simulink model "test"  (R2022b)
settings: Solver=VariableStepAuto  StartTime=0.0  StopTime=10.0  RelTol=1e-3
model workspace (MAT data in the model file):
  Var = 1
  sta = Simulink.Signal
  sta.DataType = 'Bus: Geskf_Res'
  sta.Dimensions = -1
  sta.DimensionsMode = 'auto'
  sta.Complexity = 'auto'
  sta.SampleTime = -1
  sta.SamplingMode = 'auto'
values from neighbouring files (symbols this model uses):
  a = [x1 x2]    [jocobi_test.m]
undefined symbols (not defined in the file or in its folder): stb
settings Model: Creator=89565  LastModifiedBy=89565

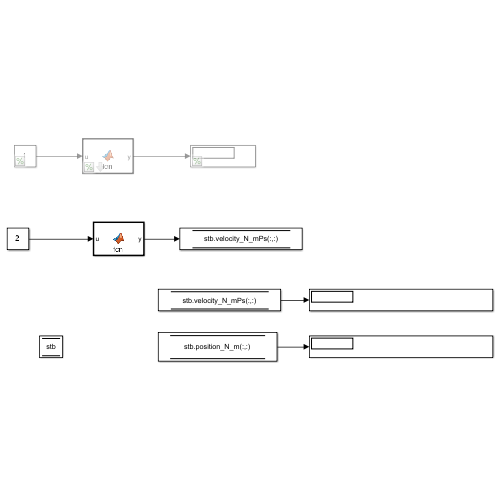
[thumbnail: Simulink's stored preview of the top-level diagram]
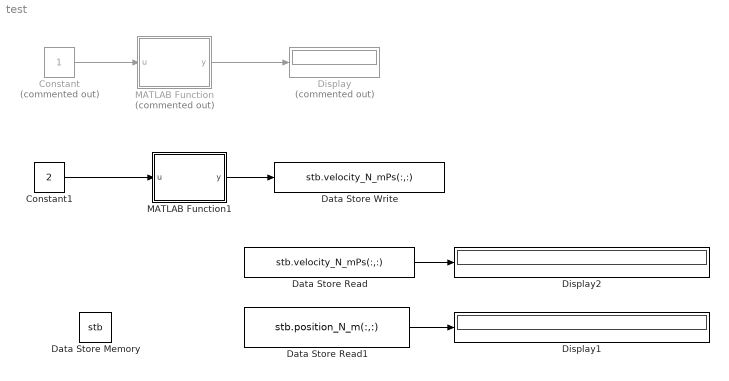
== system test ==
  Constant : Constant  Commented=on
  Constant1 : Constant  Value=2  OutDataTypeStr=double
  Data Store Read : DataStoreRead  DataStoreName=stb  DataStoreElements=stb.velocity_N_mPs(:,:)  IndexOptions=Index vector (dialog)  Indices=1  OutputSizes=1
  Data Store Read1 : DataStoreRead  DataStoreName=stb  DataStoreElements=stb.position_N_m(:,:)  IndexOptions=Index vector (dialog)  Indices=1  OutputSizes=1
  Data Store Write : DataStoreWrite  DataStoreName=stb  DataStoreElements=stb.velocity_N_mPs(:,:)  IndexOptions=Index vector (dialog)  Indices=1  OutputSizes=1
  Data Store Memory : DataStoreMemory  DataStoreName=stb  WriteAfterWriteMsg=warning  InitialValue=stb_init  ShowAdditionalParam=off  OutDataTypeStr=Bus: Geskf_Res  Dimensions=1
  Display : Display  Commented=on
  Display1 : Display
  Display2 : Display
  MATLAB Function : MATLAB Function  Commented=on  TreatAsAtomicUnit=on  mask{a=a}
  MATLAB Function1 : MATLAB Function  TreatAsAtomicUnit=on
  wires:
  Constant/1 -> MATLAB Function/1(u)
  MATLAB Function/1(y) -> Display/1
  Constant1/1 -> MATLAB Function1/1(u)
  Data Store Read/1 -> Display2/1
  Data Store Read1/1 -> Display1/1
  MATLAB Function1/1(y) -> Data Store Write/1

== matlab function test/MATLAB Function ==
  data: u input; y output; a parameter
function y = fcn(u,a)

y = u / a ;

assignin('base','a',y)

== matlab function test/MATLAB Function1 ==
  data: u input; stb data_store_memory; y output
function y = fcn(u)

y = u*single([1 1 1]');

stb.position_N_m = stb.velocity_N_mPs;

a = single(1);
